simulink model "ad3ab5cgoodnew"  (Simulink 5.0)
settings: Solver=ode45  SolverMode=SingleTasking  StartTime=0.0  StopTime=1  RelTol=1e-3  AbsTol=1e-3
CloseFcn:
  | ;slview('closediagram',bdroot);
settings Model: LastModifiedBy=Âlue Phoenix  LimitDataPoints=off  BlockReductionOpt=off  BooleanDataType=off

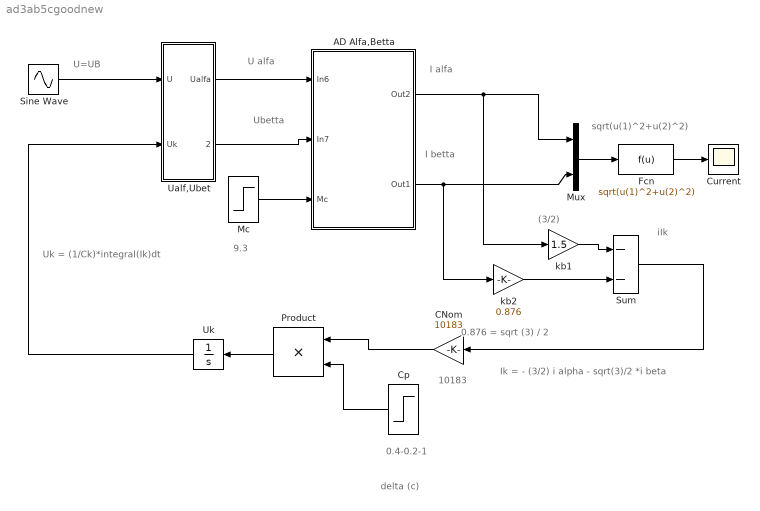
== system ad3ab5cgoodnew ==
  note: I alfa
  note: I betta
  note: U alfa
  note: Ubetta
  note: iIk
  note: U=UB
  note: Uk = (1/Ck)*integral(Ik)dt
  note: 9.3
  note: (3/2)
  note: 10183
  note: 0.4-0.2-1
  note: sqrt(u(1)^2+u(2)^2)
  note: 0.876 = sqrt (3) / 2
  note: Ik = - (3/2) i alpha - sqrt(3)/2 *i beta
  note: delta (c)
  AD Alfa,Betta : Subsystem
  CNom : Gain  Orientation=left  Gain=10183  SaturateOnIntegerOverflow=on
  Cp : Step  Orientation=left  Time=0.4  Before=0.2  SampleTime=0
  Current : Scope
      settings: TickLabels=on  TimeRange=0.2  YMin=-25000  YMax=250000  SaveName=ScopeData2  DataFormat=Array
  Fcn : Fcn  Expr=sqrt(u(1)^2+u(2)^2)
  Mc : Step  Time=0.3  After=9.3  SampleTime=0
  Mux : Mux  Inputs=2
  Product : Product  Orientation=left  SaturateOnIntegerOverflow=on  InputSameDT=on
  Sine Wave : Sin  Amplitude=311  Frequency=314  SampleTime=0
  Sum : Sum  Inputs=--  SaturateOnIntegerOverflow=on  InputSameDT=on
  Ualf,Ubet : Subsystem
  Uk : Integrator  Orientation=left
  kb1 : Gain  Gain=1.5  SaturateOnIntegerOverflow=on
  kb2 : Gain  Gain=0.876  SaturateOnIntegerOverflow=on
  wires:
  Ualf,Ubet/1(Ualfa) -> AD Alfa,Betta/1(In6)
  Ualf,Ubet/2(Ubetta) -> AD Alfa,Betta/2(In7)
  Mux/1 -> Fcn/1
  AD Alfa,Betta/1(Out2) -> Mux/1, kb1/1
  Fcn/1 -> Current/1
  AD Alfa,Betta/2(Out1) -> Mux/2, kb2/1
  Sine Wave/1 -> Ualf,Ubet/1(U)
  Uk/1 -> Ualf,Ubet/2(Uk)
  Mc/1 -> AD Alfa,Betta/3(Mc)
  Product/1 -> Uk/1
  CNom/1 -> Product/1
  Cp/1 -> Product/2
  kb1/1 -> Sum/1
  kb2/1 -> Sum/2
  Sum/1 -> CNom/1

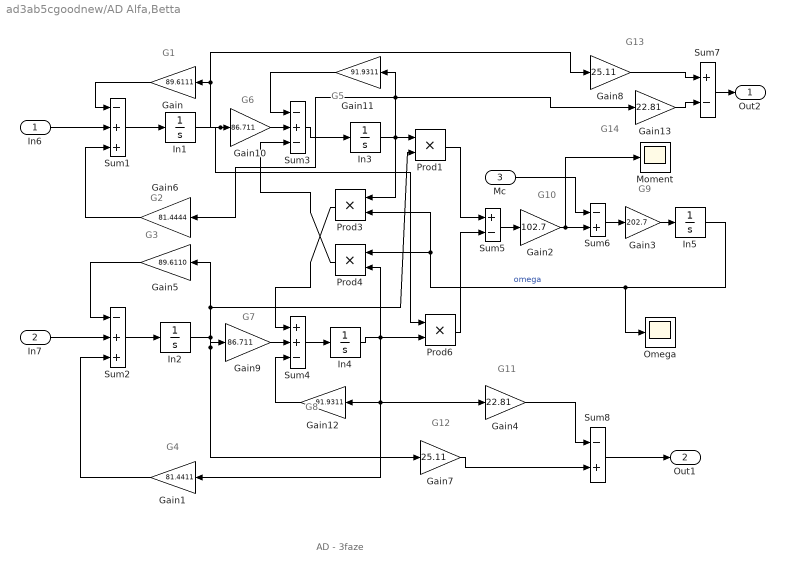
== system ad3ab5cgoodnew/AD Alfa,Betta ==
  note: G1
  note: G2
  note: G3
  note: G4
  note: G10
  note: G9
  note: G6
  note: G7
  note: G8
  note: G5
  note: AD - 3faze
  note: G14
  note: G12
  note: G13
  note: G11
  In6 : Inport
  In7 : Inport  Port=2
  Mc : Inport  Port=3
  "  Prod1" : Product  SaturateOnIntegerOverflow=on  InputSameDT=on
  Gain : Gain  Orientation=left  Gain=89.6111  SaturateOnIntegerOverflow=on
  Gain1 : Gain  Orientation=left  Gain=81.4411  SaturateOnIntegerOverflow=on
  Gain10 : Gain  Gain=86.711  SaturateOnIntegerOverflow=on
  Gain11 : Gain  Orientation=left  Gain=91.9311  SaturateOnIntegerOverflow=on
  Gain12 : Gain  Orientation=left  Gain=91.9311  SaturateOnIntegerOverflow=on
  Gain13 : Gain  Gain=22.81  SaturateOnIntegerOverflow=on
  Gain2 : Gain  Gain=102.7  SaturateOnIntegerOverflow=on
  Gain3 : Gain  Gain=202.7  SaturateOnIntegerOverflow=on
  Gain4 : Gain  Gain=22.81  SaturateOnIntegerOverflow=on
  Gain5 : Gain  Orientation=left  Gain=89.6110  SaturateOnIntegerOverflow=on
  Gain6 : Gain  Orientation=left  Gain=81.4444  SaturateOnIntegerOverflow=on
  Gain7 : Gain  Gain=25.11  SaturateOnIntegerOverflow=on
  Gain8 : Gain  Gain=25.11  SaturateOnIntegerOverflow=on
  Gain9 : Gain  Gain=86.711  SaturateOnIntegerOverflow=on
  In{1..5} (5 alike) : Integrator
  Moment : Scope
      settings: TickLabels=on  TimeRange=80  YMin=-1  YMax=2  DataFormat=Array
  Omega : Scope
      settings: TickLabels=on  TimeRange=0.2  YMin=-100  YMax=125  DataFormat=Array
  Prod3 : Product  Orientation=left  SaturateOnIntegerOverflow=on  InputSameDT=on
  Prod4 : Product  Orientation=left  SaturateOnIntegerOverflow=on  InputSameDT=on
  Prod6 : Product  SaturateOnIntegerOverflow=on  InputSameDT=on
  Sum1 : Sum  Inputs=-++  SaturateOnIntegerOverflow=on  InputSameDT=on
  Sum2 : Sum  Inputs=-++  SaturateOnIntegerOverflow=on  InputSameDT=on
  Sum3 : Sum  Inputs=-+-  SaturateOnIntegerOverflow=on  InputSameDT=on
  Sum4 : Sum  Inputs=++-  SaturateOnIntegerOverflow=on  InputSameDT=on
  Sum5 : Sum  Inputs=+-  SaturateOnIntegerOverflow=on  InputSameDT=on
  Sum6 : Sum  Inputs=-+  SaturateOnIntegerOverflow=on  InputSameDT=on
  Sum7 : Sum  Inputs=+-  SaturateOnIntegerOverflow=on  InputSameDT=on
  Sum8 : Sum  Inputs=-+  SaturateOnIntegerOverflow=on  InputSameDT=on
  Out2 : Outport
  Out1 : Outport  Port=2
  wires:
  Gain/1 -> Sum1/1
  Sum2/1 -> In2/1
  In4/1 -> Prod4/2, Prod6/2, Gain1/1, Gain12/1, Gain4/1
  In3/1 -> Prod3/1, "  Prod1"/1, Gain6/1, Gain11/1, Gain13/1
  Prod6/1 -> Sum5/2
  Sum6/1 -> Gain3/1
  Gain3/1 -> In5/1
  "  Prod1"/1 -> Sum5/1
  Sum3/1 -> In3/1
  Sum5/1 -> Gain2/1
  Sum1/1 -> In1/1
  In2/1 -> "  Prod1"/2, Gain5/1, Gain9/1, Gain7/1
  In1/1 -> Gain10/1, Gain/1, Gain8/1, Prod6/1
  Gain10/1 -> Sum3/2
  Gain9/1 -> Sum4/2
  Gain5/1 -> Sum2/1
  Prod4/1 -> Sum3/3
  Prod3/1 -> Sum4/1
  Gain2/1 -> Sum6/2, Moment/1
  Gain11/1 -> Sum3/1
  Gain12/1 -> Sum4/3
  In5/1 -> Prod3/2, Prod4/1, Omega/1  "omega"
  Sum4/1 -> In4/1
  Gain7/1 -> Sum8/2
  Gain4/1 -> Sum8/1
  Gain6/1 -> Sum1/3
  Gain1/1 -> Sum2/3
  In7/1 -> Sum2/2
  Gain8/1 -> Sum7/1
  Gain13/1 -> Sum7/2
  In6/1 -> Sum1/2
  Sum8/1 -> Out1/1
  Sum7/1 -> Out2/1
  Mc/1 -> Sum6/1

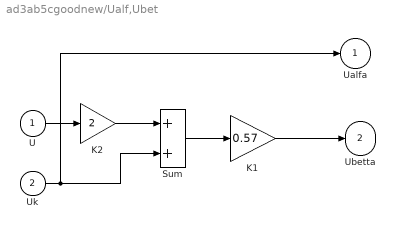
== system ad3ab5cgoodnew/Ualf,Ubet ==
  U : Inport
  Uk : Inport  Port=2
  K1 : Gain  Gain=0.57  SaturateOnIntegerOverflow=on
  K2 : Gain  Gain=2  SaturateOnIntegerOverflow=on
  Sum : Sum  SaturateOnIntegerOverflow=on  InputSameDT=on
  Ualfa : Outport
  Ubetta : Outport  Port=2
  wires:
  K1/1 -> Ubetta/1
  Sum/1 -> K1/1
  Uk/1 -> Sum/2, Ualfa/1
  U/1 -> K2/1
  K2/1 -> Sum/1
